simulink model "Grua_MC_R2_Ciclo_Completo_SFC"  (R2025b)
settings: Solver=ode23t  StartTime=0.0  StopTime=640  MaxStep=T_s  RelTol=1e-4
InitFcn:
  | addpath(fileparts(get_param(bdroot,'FileName')),'-begin');
  | run(fullfile(fileparts(get_param(bdroot,'FileName')),'definir_buses_variadores.m'));
  | run(fullfile(fileparts(get_param(bdroot,'FileName')),'parametros_ganancias_cascada_29072026.m'));
  | run(fullfile(fileparts(get_param(bdroot,'FileName')),'configurar_modelo_final_hmi.m'));
  | run(fullfile(fileparts(get_param(bdroot,'FileName')),'configurar_parametros_variadores.m'));
  | Pvis.Ts_viz=.04;Pvis.enable=true;Pvis.keepFigureOnTerminate=true;Pvis.hmi.fastDiagnostic=false;
undefined symbols (not defined in the file or in its folder): b_cx, b_cy, b_hb, b_hEb, b_heq, b_t, b_tb, b_teq, b_tw, b_wu, g, H_c, HMI, i_h, i_t, J_heq, J_teq, K_cy, K_tw, k_wu, L_h0, l_hi, M_c_profile, M_s, M_t, MC_FF, nLevels0, omega_hmRATED, r_hd, r_td, slotBlock, T_hbMax, T_hEbMax, T_hmMax, T_s, T_s1, T_tbMax, T_tmMax, tau_hm, tau_tm, traj_duration, traj_x_start, traj_x_target, v_hmaxLoaded, v_hmaxUnloaded, x_tmax, x_tmin, Y_c0, Y_t0, Zbase
libraries: simulink x1, aerolibanimutils x1
(part 2 of 4)

== system Grua_MC_R2_Ciclo_Completo_SFC/Actualizar_Yc ==
  tipo_evento : Inport
  slot_evento : Inport  Port=2
  Trigger : TriggerPort  VariantControl=(inherit)  PortDimensions=1
  Constant : Constant  Value=Zbase
  Constant1 : Constant  Value=slotBlock
  Constant2 : Constant  Value=H_c
  Unit Delay : UnitDelay  InitialCondition=nLevels0  SampleTime=-1  HasFrameUpgradeWarning=on
  update_perfil_std : MATLAB Function  TreatAsAtomicUnit=on
  Y_c : Outport  InitialOutput=Y_c0
  wires:
  update_perfil_std/2(Y_c) -> Y_c/1
  slot_evento/1 -> update_perfil_std/3(slot_evento)
  update_perfil_std/1(nLevels_new) -> Unit Delay/1
  tipo_evento/1 -> update_perfil_std/2(tipo_evento)
  Unit Delay/1 -> update_perfil_std/1(nLevels)
  Constant/1 -> update_perfil_std/4(Zbase)
  Constant1/1 -> update_perfil_std/5(slotBlock)
  Constant2/1 -> update_perfil_std/6(h_std)

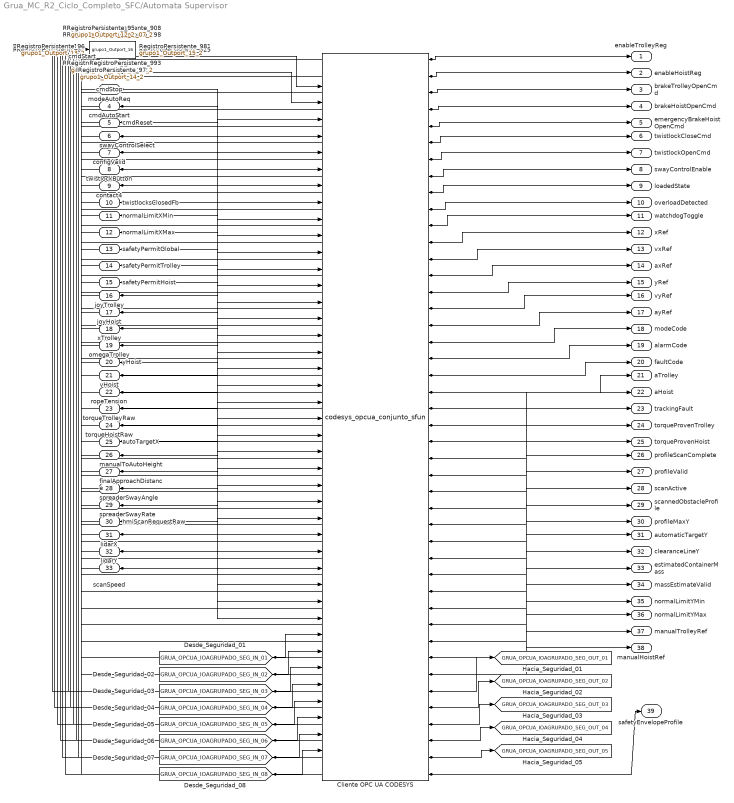
== system Grua_MC_R2_Ciclo_Completo_SFC/Automata Supervisor ==
  cmdStart : Inport
  cmdStop : Inport  Port=2
  modeAutoReq : Inport  Port=3
  cmdAutoStart : Inport  Port=4
  cmdReset : Inport  Port=5
  swayControlSelect : Inport  Port=6
  configValid : Inport  Port=7
  twistlockButton : Inport  Port=8
  contact4 : Inport  Port=9
  twistlocksClosedFb : Inport  Port=10
  normalLimitXMin : Inport  Port=11
  normalLimitXMax : Inport  Port=12
  safetyPermitGlobal : Inport  Port=13
  safetyPermitTrolley : Inport  Port=14
  safetyPermitHoist : Inport  Port=15
  joyTrolley : Inport  Port=16
  joyHoist : Inport  Port=17
  xTrolley : Inport  Port=18
  omegaTrolley : Inport  Port=19
  yHoist : Inport  Port=20
  vHoist : Inport  Port=21
  ropeTension : Inport  Port=22
  torqueTrolleyRaw : Inport  Port=23
  torqueHoistRaw : Inport  Port=24
  autoTargetX : Inport  Port=25
  manualToAutoHeight : Inport  Port=26
  finalApproachDistance : Inport  Port=27
  spreaderSwayAngle : Inport  Port=28
  spreaderSwayRate : Inport  Port=29
  hmiScanRequestRaw : Inport  Port=30
  lidarX : Inport  Port=31
  lidarY : Inport  Port=32
  scanSpeed : Inport  Port=33
  Cliente OPC UA CODESYS : M-S-Function  FunctionName=codesys_opcua_conjunto_sfun
  RegistroPersistente_100 : ToWorkspace  VariableName=grupo1_Outport_17  SaveFormat=Timeseries  SampleTime=-1
      settings: Decimation=10
  RegistroPersistente_101 : ToWorkspace  VariableName=grupo1_Outport_18_2  SaveFormat=Timeseries  SampleTime=-1
      settings: Decimation=10
  RegistroPersistente_102 : ToWorkspace  VariableName=grupo1_Outport_19_2  SaveFormat=Timeseries  SampleTime=-1
      settings: Decimation=10
  RegistroPersistente_103 : ToWorkspace  VariableName=grupo1_Outport_20_2  SaveFormat=Timeseries  SampleTime=-1
      settings: Decimation=10
  RegistroPersistente_104 : ToWorkspace  VariableName=grupo1_Outport_21_2  SaveFormat=Timeseries  SampleTime=-1
      settings: Decimation=10
  RegistroPersistente_105 : ToWorkspace  VariableName=grupo1_Outport_22_2  SaveFormat=Timeseries  SampleTime=-1
      settings: Decimation=10
  RegistroPersistente_106 : ToWorkspace  VariableName=grupo1_Outport_23_2  SaveFormat=Timeseries  SampleTime=-1
      settings: Decimation=10
  RegistroPersistente_107 : ToWorkspace  VariableName=grupo1_Outport_24_2  SaveFormat=Timeseries  SampleTime=-1
      settings: Decimation=10
  RegistroPersistente_108 : ToWorkspace  VariableName=grupo1_Outport_25_2  SaveFormat=Timeseries  SampleTime=-1
      settings: Decimation=10
  RegistroPersistente_109 : ToWorkspace  VariableName=grupo1_Outport_26_2  SaveFormat=Timeseries  SampleTime=-1
      settings: Decimation=10
  RegistroPersistente_110 : ToWorkspace  VariableName=grupo1_Outport_27_2  SaveFormat=Timeseries  SampleTime=-1
      settings: Decimation=10
  RegistroPersistente_111 : ToWorkspace  VariableName=grupo1_Outport_28_2  SaveFormat=Timeseries  SampleTime=-1
      settings: Decimation=10
  RegistroPersistente_112 : ToWorkspace  VariableName=grupo1_Outport_29_2  SaveFormat=Timeseries  SampleTime=-1
      settings: Decimation=10
  RegistroPersistente_113 : ToWorkspace  VariableName=grupo1_Outport_30_2  SaveFormat=Timeseries  SampleTime=-1
      settings: Decimation=10
  RegistroPersistente_114 : ToWorkspace  VariableName=grupo1_Outport_31_2  SaveFormat=Timeseries  SampleTime=-1
      settings: Decimation=10
  RegistroPersistente_115 : ToWorkspace  VariableName=grupo1_Outport_32_2  SaveFormat=Timeseries  SampleTime=-1
      settings: Decimation=10
  RegistroPersistente_116 : ToWorkspace  VariableName=grupo1_Outport_33_2  SaveFormat=Timeseries  SampleTime=-1
      settings: Decimation=10
  RegistroPersistente_117 : ToWorkspace  VariableName=grupo1_Outport_34_2  SaveFormat=Timeseries  SampleTime=-1
      settings: Decimation=10
  RegistroPersistente_118 : ToWorkspace  VariableName=grupo1_Outport_35_2  SaveFormat=Timeseries  SampleTime=-1
      settings: Decimation=10
  RegistroPersistente_119 : ToWorkspace  VariableName=grupo1_Outport_36_2  SaveFormat=Timeseries  SampleTime=-1
      settings: Decimation=10
  RegistroPersistente_120 : ToWorkspace  VariableName=grupo1_Outport_37_2  SaveFormat=Timeseries  SampleTime=-1
      settings: Decimation=10
  RegistroPersistente_121 : ToWorkspace  VariableName=grupo1_Outport_38_2  SaveFormat=Timeseries  SampleTime=-1
      settings: Decimation=10
  RegistroPersistente_122 : ToWorkspace  VariableName=grupo1_Outport_39  SaveFormat=Timeseries  SampleTime=-1
      settings: Decimation=10
  RegistroPersistente_123 : ToWorkspace  VariableName=grupo1_Outport_40  SaveFormat=Timeseries  SampleTime=-1
      settings: Decimation=10
  RegistroPersistente_124 : ToWorkspace  VariableName=grupo1_Outport_41  SaveFormat=Timeseries  SampleTime=-1
      settings: Decimation=10
  RegistroPersistente_125 : ToWorkspace  VariableName=grupo1_Outport_42  SaveFormat=Timeseries  SampleTime=-1
      settings: Decimation=10
  RegistroPersistente_126 : ToWorkspace  VariableName=grupo1_Outport_43  SaveFormat=Timeseries  SampleTime=-1
      settings: Decimation=10
  RegistroPersistente_127 : ToWorkspace  VariableName=grupo1_Outport_44  SaveFormat=Timeseries  SampleTime=-1
      settings: Decimation=10
  RegistroPersistente_128 : ToWorkspace  VariableName=grupo1_Inport_34  SaveFormat=Timeseries  SampleTime=-1
      settings: Decimation=10
  RegistroPersistente_129 : ToWorkspace  VariableName=grupo1_Inport_35  SaveFormat=Timeseries  SampleTime=-1
      settings: Decimation=10
  RegistroPersistente_130 : ToWorkspace  VariableName=grupo1_Inport_36  SaveFormat=Timeseries  SampleTime=-1
      settings: Decimation=10
  RegistroPersistente_131 : ToWorkspace  VariableName=grupo1_Inport_37  SaveFormat=Timeseries  SampleTime=-1
      settings: Decimation=10
  RegistroPersistente_132 : ToWorkspace  VariableName=grupo1_Inport_38  SaveFormat=Timeseries  SampleTime=-1
      settings: Decimation=10
  RegistroPersistente_133 : ToWorkspace  VariableName=grupo1_Inport_39  SaveFormat=Timeseries  SampleTime=-1
      settings: Decimation=10
  RegistroPersistente_134 : ToWorkspace  VariableName=grupo1_Inport_40  SaveFormat=Timeseries  SampleTime=-1
      settings: Decimation=10
  RegistroPersistente_135 : ToWorkspace  VariableName=grupo1_Inport_41  SaveFormat=Timeseries  SampleTime=-1
      settings: Decimation=10
  RegistroPersistente_51 : ToWorkspace  VariableName=grupo1_Inport_01_2  SaveFormat=Timeseries  SampleTime=-1
      settings: Decimation=10
  RegistroPersistente_52 : ToWorkspace  VariableName=grupo1_Inport_02_2  SaveFormat=Timeseries  SampleTime=-1
      settings: Decimation=10
  RegistroPersistente_53 : ToWorkspace  VariableName=grupo1_Inport_03_2  SaveFormat=Timeseries  SampleTime=-1
      settings: Decimation=10
  RegistroPersistente_54 : ToWorkspace  VariableName=grupo1_Inport_04_2  SaveFormat=Timeseries  SampleTime=-1
      settings: Decimation=10
  RegistroPersistente_55 : ToWorkspace  VariableName=grupo1_Inport_05_2  SaveFormat=Timeseries  SampleTime=-1
      settings: Decimation=10
  RegistroPersistente_56 : ToWorkspace  VariableName=grupo1_Inport_06_2  SaveFormat=Timeseries  SampleTime=-1
      settings: Decimation=10
  RegistroPersistente_57 : ToWorkspace  VariableName=grupo1_Inport_07_2  SaveFormat=Timeseries  SampleTime=-1
      settings: Decimation=10
  RegistroPersistente_58 : ToWorkspace  VariableName=grupo1_Inport_08_2  SaveFormat=Timeseries  SampleTime=-1
      settings: Decimation=10
  RegistroPersistente_59 : ToWorkspace  VariableName=grupo1_Inport_09_2  SaveFormat=Timeseries  SampleTime=-1
      settings: Decimation=10
  RegistroPersistente_60 : ToWorkspace  VariableName=grupo1_Inport_10_2  SaveFormat=Timeseries  SampleTime=-1
      settings: Decimation=10
  RegistroPersistente_61 : ToWorkspace  VariableName=grupo1_Inport_11_2  SaveFormat=Timeseries  SampleTime=-1
      settings: Decimation=10
  RegistroPersistente_62 : ToWorkspace  VariableName=grupo1_Inport_12_2  SaveFormat=Timeseries  SampleTime=-1
      settings: Decimation=10
  RegistroPersistente_63 : ToWorkspace  VariableName=grupo1_Inport_13_2  SaveFormat=Timeseries  SampleTime=-1
      settings: Decimation=10
  RegistroPersistente_64 : ToWorkspace  VariableName=grupo1_Inport_14_2  SaveFormat=Timeseries  SampleTime=-1
      settings: Decimation=10
  RegistroPersistente_65 : ToWorkspace  VariableName=grupo1_Inport_15_2  SaveFormat=Timeseries  SampleTime=-1
      settings: Decimation=10
  RegistroPersistente_66 : ToWorkspace  VariableName=grupo1_Inport_16_2  SaveFormat=Timeseries  SampleTime=-1
      settings: Decimation=10
  RegistroPersistente_67 : ToWorkspace  VariableName=grupo1_Inport_17_2  SaveFormat=Timeseries  SampleTime=-1
      settings: Decimation=10
  RegistroPersistente_68 : ToWorkspace  VariableName=grupo1_Inport_18_2  SaveFormat=Timeseries  SampleTime=-1
      settings: Decimation=10
  RegistroPersistente_69 : ToWorkspace  VariableName=grupo1_Inport_19_2  SaveFormat=Timeseries  SampleTime=-1
      settings: Decimation=10
  RegistroPersistente_70 : ToWorkspace  VariableName=grupo1_Inport_20_2  SaveFormat=Timeseries  SampleTime=-1
      settings: Decimation=10
  RegistroPersistente_71 : ToWorkspace  VariableName=grupo1_Inport_21_2  SaveFormat=Timeseries  SampleTime=-1
      settings: Decimation=10
  RegistroPersistente_72 : ToWorkspace  VariableName=grupo1_Inport_22_2  SaveFormat=Timeseries  SampleTime=-1
      settings: Decimation=10
  RegistroPersistente_73 : ToWorkspace  VariableName=grupo1_Inport_23_2  SaveFormat=Timeseries  SampleTime=-1
      settings: Decimation=10
  RegistroPersistente_74 : ToWorkspace  VariableName=grupo1_Inport_24_2  SaveFormat=Timeseries  SampleTime=-1
      settings: Decimation=10
  RegistroPersistente_75 : ToWorkspace  VariableName=grupo1_Inport_25_2  SaveFormat=Timeseries  SampleTime=-1
      settings: Decimation=10
  RegistroPersistente_76 : ToWorkspace  VariableName=grupo1_Inport_26_2  SaveFormat=Timeseries  SampleTime=-1
      settings: Decimation=10
  RegistroPersistente_77 : ToWorkspace  VariableName=grupo1_Inport_27_2  SaveFormat=Timeseries  SampleTime=-1
      settings: Decimation=10
  RegistroPersistente_78 : ToWorkspace  VariableName=grupo1_Inport_28_2  SaveFormat=Timeseries  SampleTime=-1
      settings: Decimation=10
  RegistroPersistente_79 : ToWorkspace  VariableName=grupo1_Inport_29_2  SaveFormat=Timeseries  SampleTime=-1
      settings: Decimation=10
  RegistroPersistente_80 : ToWorkspace  VariableName=grupo1_Inport_30_2  SaveFormat=Timeseries  SampleTime=-1
      settings: Decimation=10
  RegistroPersistente_81 : ToWorkspace  VariableName=grupo1_Inport_31_2  SaveFormat=Timeseries  SampleTime=-1
      settings: Decimation=10
  RegistroPersistente_82 : ToWorkspace  VariableName=grupo1_Inport_32_2  SaveFormat=Timeseries  SampleTime=-1
      settings: Decimation=10
  RegistroPersistente_83 : ToWorkspace  VariableName=grupo1_Inport_33_2  SaveFormat=Timeseries  SampleTime=-1
      settings: Decimation=10
  RegistroPersistente_84 : ToWorkspace  VariableName=grupo1_Outport_01_2  SaveFormat=Timeseries  SampleTime=-1
      settings: Decimation=10
  RegistroPersistente_85 : ToWorkspace  VariableName=grupo1_Outport_02_2  SaveFormat=Timeseries  SampleTime=-1
      settings: Decimation=10
  RegistroPersistente_86 : ToWorkspace  VariableName=grupo1_Outport_03  SaveFormat=Timeseries  SampleTime=-1
      settings: Decimation=10
  RegistroPersistente_87 : ToWorkspace  VariableName=grupo1_Outport_04_2  SaveFormat=Timeseries  SampleTime=-1
      settings: Decimation=10
  RegistroPersistente_88 : ToWorkspace  VariableName=grupo1_Outport_05_2  SaveFormat=Timeseries  SampleTime=-1
      settings: Decimation=10
  RegistroPersistente_89 : ToWorkspace  VariableName=grupo1_Outport_06_2  SaveFormat=Timeseries  SampleTime=-1
      settings: Decimation=10
  RegistroPersistente_90 : ToWorkspace  VariableName=grupo1_Outport_07_2  SaveFormat=Timeseries  SampleTime=-1
      settings: Decimation=10
  RegistroPersistente_91 : ToWorkspace  VariableName=grupo1_Outport_08  SaveFormat=Timeseries  SampleTime=-1
      settings: Decimation=10
  RegistroPersistente_92 : ToWorkspace  VariableName=grupo1_Outport_09_2  SaveFormat=Timeseries  SampleTime=-1
      settings: Decimation=10
  RegistroPersistente_93 : ToWorkspace  VariableName=grupo1_Outport_10_2  SaveFormat=Timeseries  SampleTime=-1
      settings: Decimation=10
  RegistroPersistente_94 : ToWorkspace  VariableName=grupo1_Outport_11_2  SaveFormat=Timeseries  SampleTime=-1
      settings: Decimation=10
  RegistroPersistente_95 : ToWorkspace  VariableName=grupo1_Outport_12_2  SaveFormat=Timeseries  SampleTime=-1
      settings: Decimation=10
  RegistroPersistente_96 : ToWorkspace  VariableName=grupo1_Outport_13_2  SaveFormat=Timeseries  SampleTime=-1
      settings: Decimation=10
  RegistroPersistente_97 : ToWorkspace  VariableName=grupo1_Outport_14_2  SaveFormat=Timeseries  SampleTime=-1
      settings: Decimation=10
  RegistroPersistente_98 : ToWorkspace  VariableName=grupo1_Outport_15_2  SaveFormat=Timeseries  SampleTime=-1
      settings: Decimation=10
  RegistroPersistente_99 : ToWorkspace  VariableName=grupo1_Outport_16  SaveFormat=Timeseries  SampleTime=-1
      settings: Decimation=10
  enableTrolleyReg : Outport
  enableHoistReg : Outport  Port=2
  brakeTrolleyOpenCmd : Outport  Port=3
  brakeHoistOpenCmd : Outport  Port=4
  emergencyBrakeHoistOpenCmd : Outport  Port=5
  twistlockCloseCmd : Outport  Port=6
  twistlockOpenCmd : Outport  Port=7
  swayControlEnable : Outport  Port=8
  loadedState : Outport  Port=9
  overloadDetected : Outport  Port=10
  watchdogToggle : Outport  Port=11
  xRef : Outport  Port=12
  vxRef : Outport  Port=13
  axRef : Outport  Port=14
  yRef : Outport  Port=15
  vyRef : Outport  Port=16
  ayRef : Outport  Port=17
  modeCode : Outport  Port=18
  alarmCode : Outport  Port=19
  faultCode : Outport  Port=20
  aTrolley : Outport  Port=21
  aHoist : Outport  Port=22
  trackingFault : Outport  Port=23
  torqueProvenTrolley : Outport  Port=24
  torqueProvenHoist : Outport  Port=25
  profileScanComplete : Outport  Port=26
  profileValid : Outport  Port=27
  scanActive : Outport  Port=28
  scannedObstacleProfile : Outport  Port=29
  profileMaxY : Outport  Port=30
  automaticTargetY : Outport  Port=31
  clearanceLineY : Outport  Port=32
  estimatedContainerMass : Outport  Port=33
  massEstimateValid : Outport  Port=34
  normalLimitYMin : Outport  Port=35
  normalLimitYMax : Outport  Port=36
  manualTrolleyRef : Outport  Port=37
  manualHoistRef : Outport  Port=38
  safetyEnvelopeProfile : Outport  Port=39
  tag scope: GRUA_OPCUA_IOAGRUPADO_SEG_OUT_01=global, GRUA_OPCUA_IOAGRUPADO_SEG_OUT_02=global, GRUA_OPCUA_IOAGRUPADO_SEG_OUT_03=global, GRUA_OPCUA_IOAGRUPADO_SEG_OUT_04=global, GRUA_OPCUA_IOAGRUPADO_SEG_OUT_05=global
  wires:
  Cliente OPC UA CODESYS/44 -> safetyEnvelopeProfile/1, RegistroPersistente_127/1
  Cliente OPC UA CODESYS/43 -> [GRUA_OPCUA_IOAGRUPADO_SEG_OUT_05], RegistroPersistente_126/1
  Cliente OPC UA CODESYS/42 -> [GRUA_OPCUA_IOAGRUPADO_SEG_OUT_04], RegistroPersistente_125/1
  Cliente OPC UA CODESYS/41 -> [GRUA_OPCUA_IOAGRUPADO_SEG_OUT_03], RegistroPersistente_124/1
  Cliente OPC UA CODESYS/40 -> [GRUA_OPCUA_IOAGRUPADO_SEG_OUT_02], RegistroPersistente_123/1
  Cliente OPC UA CODESYS/39 -> [GRUA_OPCUA_IOAGRUPADO_SEG_OUT_01], RegistroPersistente_122/1
  [GRUA_OPCUA_IOAGRUPADO_SEG_IN_08] -> Cliente OPC UA CODESYS/41, RegistroPersistente_135/1
  [GRUA_OPCUA_IOAGRUPADO_SEG_IN_07] -> Cliente OPC UA CODESYS/40, RegistroPersistente_134/1
  [GRUA_OPCUA_IOAGRUPADO_SEG_IN_06] -> Cliente OPC UA CODESYS/39, RegistroPersistente_133/1
  [GRUA_OPCUA_IOAGRUPADO_SEG_IN_05] -> Cliente OPC UA CODESYS/38, RegistroPersistente_132/1
  [GRUA_OPCUA_IOAGRUPADO_SEG_IN_04] -> Cliente OPC UA CODESYS/37, RegistroPersistente_131/1
  [GRUA_OPCUA_IOAGRUPADO_SEG_IN_03] -> Cliente OPC UA CODESYS/36, RegistroPersistente_130/1
  [GRUA_OPCUA_IOAGRUPADO_SEG_IN_02] -> Cliente OPC UA CODESYS/35, RegistroPersistente_129/1
  [GRUA_OPCUA_IOAGRUPADO_SEG_IN_01] -> Cliente OPC UA CODESYS/34, RegistroPersistente_128/1
  Cliente OPC UA CODESYS/38 -> manualHoistRef/1, RegistroPersistente_121/1
  Cliente OPC UA CODESYS/37 -> manualTrolleyRef/1, RegistroPersistente_120/1
  Cliente OPC UA CODESYS/36 -> normalLimitYMax/1, RegistroPersistente_119/1
  Cliente OPC UA CODESYS/35 -> normalLimitYMin/1, RegistroPersistente_118/1
  Cliente OPC UA CODESYS/34 -> massEstimateValid/1, RegistroPersistente_117/1
  Cliente OPC UA CODESYS/33 -> estimatedContainerMass/1, RegistroPersistente_116/1
  Cliente OPC UA CODESYS/32 -> clearanceLineY/1, RegistroPersistente_115/1
  Cliente OPC UA CODESYS/31 -> automaticTargetY/1, RegistroPersistente_114/1
  Cliente OPC UA CODESYS/30 -> profileMaxY/1, RegistroPersistente_113/1
  Cliente OPC UA CODESYS/29 -> scannedObstacleProfile/1, RegistroPersistente_112/1
  Cliente OPC UA CODESYS/28 -> scanActive/1, RegistroPersistente_111/1
  Cliente OPC UA CODESYS/27 -> profileValid/1, RegistroPersistente_110/1
  Cliente OPC UA CODESYS/26 -> profileScanComplete/1, RegistroPersistente_109/1
  Cliente OPC UA CODESYS/25 -> torqueProvenHoist/1, RegistroPersistente_108/1
  Cliente OPC UA CODESYS/24 -> torqueProvenTrolley/1, RegistroPersistente_107/1
  Cliente OPC UA CODESYS/23 -> trackingFault/1, RegistroPersistente_106/1
  Cliente OPC UA CODESYS/22 -> aHoist/1, RegistroPersistente_105/1
  Cliente OPC UA CODESYS/21 -> aTrolley/1, RegistroPersistente_104/1
  Cliente OPC UA CODESYS/20 -> faultCode/1, RegistroPersistente_103/1
  Cliente OPC UA CODESYS/19 -> alarmCode/1, RegistroPersistente_102/1
  Cliente OPC UA CODESYS/18 -> modeCode/1, RegistroPersistente_101/1
  Cliente OPC UA CODESYS/17 -> ayRef/1, RegistroPersistente_100/1
  Cliente OPC UA CODESYS/16 -> vyRef/1, RegistroPersistente_99/1
  Cliente OPC UA CODESYS/15 -> yRef/1, RegistroPersistente_98/1
  Cliente OPC UA CODESYS/14 -> axRef/1, RegistroPersistente_97/1
  Cliente OPC UA CODESYS/13 -> vxRef/1, RegistroPersistente_96/1
  Cliente OPC UA CODESYS/12 -> xRef/1, RegistroPersistente_95/1
  Cliente OPC UA CODESYS/11 -> watchdogToggle/1, RegistroPersistente_94/1
  Cliente OPC UA CODESYS/10 -> overloadDetected/1, RegistroPersistente_93/1
  Cliente OPC UA CODESYS/9 -> loadedState/1, RegistroPersistente_92/1
  Cliente OPC UA CODESYS/8 -> swayControlEnable/1, RegistroPersistente_91/1
  Cliente OPC UA CODESYS/7 -> twistlockOpenCmd/1, RegistroPersistente_90/1
  Cliente OPC UA CODESYS/6 -> twistlockCloseCmd/1, RegistroPersistente_89/1
  Cliente OPC UA CODESYS/5 -> emergencyBrakeHoistOpenCmd/1, RegistroPersistente_88/1
  Cliente OPC UA CODESYS/4 -> brakeHoistOpenCmd/1, RegistroPersistente_87/1
  Cliente OPC UA CODESYS/3 -> brakeTrolleyOpenCmd/1, RegistroPersistente_86/1
  Cliente OPC UA CODESYS/2 -> enableHoistReg/1, RegistroPersistente_85/1
  Cliente OPC UA CODESYS/1 -> enableTrolleyReg/1, RegistroPersistente_84/1
  scanSpeed/1 -> Cliente OPC UA CODESYS/33, RegistroPersistente_83/1
  lidarY/1 -> Cliente OPC UA CODESYS/32, RegistroPersistente_82/1
  lidarX/1 -> Cliente OPC UA CODESYS/31, RegistroPersistente_81/1
  hmiScanRequestRaw/1 -> Cliente OPC UA CODESYS/30, RegistroPersistente_80/1
  spreaderSwayRate/1 -> Cliente OPC UA CODESYS/29, RegistroPersistente_79/1
  spreaderSwayAngle/1 -> Cliente OPC UA CODESYS/28, RegistroPersistente_78/1
  finalApproachDistance/1 -> Cliente OPC UA CODESYS/27, RegistroPersistente_77/1
  manualToAutoHeight/1 -> Cliente OPC UA CODESYS/26, RegistroPersistente_76/1
  autoTargetX/1 -> Cliente OPC UA CODESYS/25, RegistroPersistente_75/1
  torqueHoistRaw/1 -> Cliente OPC UA CODESYS/24, RegistroPersistente_74/1
  torqueTrolleyRaw/1 -> Cliente OPC UA CODESYS/23, RegistroPersistente_73/1
  ropeTension/1 -> Cliente OPC UA CODESYS/22, RegistroPersistente_72/1
  vHoist/1 -> Cliente OPC UA CODESYS/21, RegistroPersistente_71/1
  yHoist/1 -> Cliente OPC UA CODESYS/20, RegistroPersistente_70/1
  omegaTrolley/1 -> Cliente OPC UA CODESYS/19, RegistroPersistente_69/1
  xTrolley/1 -> Cliente OPC UA CODESYS/18, RegistroPersistente_68/1
  joyHoist/1 -> Cliente OPC UA CODESYS/17, RegistroPersistente_67/1
  joyTrolley/1 -> Cliente OPC UA CODESYS/16, RegistroPersistente_66/1
  safetyPermitHoist/1 -> Cliente OPC UA CODESYS/15, RegistroPersistente_65/1
  safetyPermitTrolley/1 -> Cliente OPC UA CODESYS/14, RegistroPersistente_64/1
  safetyPermitGlobal/1 -> Cliente OPC UA CODESYS/13, RegistroPersistente_63/1
  normalLimitXMax/1 -> Cliente OPC UA CODESYS/12, RegistroPersistente_62/1
  normalLimitXMin/1 -> Cliente OPC UA CODESYS/11, RegistroPersistente_61/1
  twistlocksClosedFb/1 -> Cliente OPC UA CODESYS/10, RegistroPersistente_60/1
  contact4/1 -> Cliente OPC UA CODESYS/9, RegistroPersistente_59/1
  twistlockButton/1 -> Cliente OPC UA CODESYS/8, RegistroPersistente_58/1
  configValid/1 -> Cliente OPC UA CODESYS/7, RegistroPersistente_57/1
  swayControlSelect/1 -> Cliente OPC UA CODESYS/6, RegistroPersistente_56/1
  cmdReset/1 -> Cliente OPC UA CODESYS/5, RegistroPersistente_55/1
  cmdAutoStart/1 -> Cliente OPC UA CODESYS/4, RegistroPersistente_54/1
  modeAutoReq/1 -> Cliente OPC UA CODESYS/3, RegistroPersistente_53/1
  cmdStop/1 -> Cliente OPC UA CODESYS/2, RegistroPersistente_52/1
  cmdStart/1 -> Cliente OPC UA CODESYS/1, RegistroPersistente_51/1

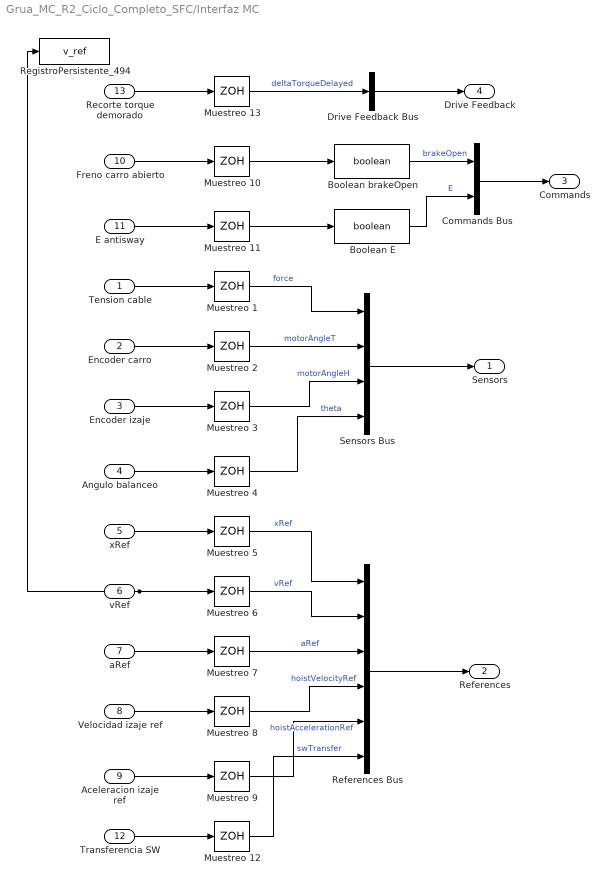
== system Grua_MC_R2_Ciclo_Completo_SFC/Interfaz MC ==
  Tension cable : Inport
  Encoder carro : Inport  Port=2
  Encoder izaje : Inport  Port=3
  Angulo balanceo : Inport  Port=4
  xRef : Inport  Port=5
  vRef : Inport  Port=6
  aRef : Inport  Port=7
  Velocidad izaje ref : Inport  Port=8
  Aceleracion izaje ref : Inport  Port=9
  Freno carro abierto : Inport  Port=10
  E antisway : Inport  Port=11
  Transferencia SW : Inport  Port=12
  Recorte torque demorado : Inport  Port=13
  Boolean E : DataTypeConversion  OutDataTypeStr=boolean  SaturateOnIntegerOverflow=off  RndMeth=Floor
  Boolean brakeOpen : DataTypeConversion  OutDataTypeStr=boolean  SaturateOnIntegerOverflow=off  RndMeth=Floor
  Commands Bus : BusCreator  Inputs=2  OutDataTypeStr=Bus: MCFF_Commands  NonVirtualBus=on
  Drive Feedback Bus : BusCreator  Inputs=1  OutDataTypeStr=Bus: MCFF_DriveFeedback  NonVirtualBus=on
  Muestreo {1..13} (13 alike) : ZeroOrderHold  SampleTime=T_s
  References Bus : BusCreator  Inputs=6  OutDataTypeStr=Bus: MCFF_References  NonVirtualBus=on
  RegistroPersistente_494 : ToWorkspace  VariableName=v_ref  SaveFormat=Timeseries  SampleTime=-1
      settings: Decimation=10
  Sensors Bus : BusCreator  Inputs=4  OutDataTypeStr=Bus: MCFF_Sensors  NonVirtualBus=on
  Sensors : Outport
  References : Outport  Port=2
  Commands : Outport  Port=3
  Drive Feedback : Outport  Port=4
  wires:
  Drive Feedback Bus/1 -> Drive Feedback/1
  Muestreo 4/1 -> Sensors Bus/4  "theta"
  E antisway/1 -> Muestreo 11/1
  Recorte torque demorado/1 -> Muestreo 13/1
  Encoder carro/1 -> Muestreo 2/1
  Tension cable/1 -> Muestreo 1/1
  Muestreo 3/1 -> Sensors Bus/3  "motorAngleH"
  Freno carro abierto/1 -> Muestreo 10/1
  xRef/1 -> Muestreo 5/1
  Angulo balanceo/1 -> Muestreo 4/1
  Muestreo 11/1 -> Boolean E/1
  Encoder izaje/1 -> Muestreo 3/1
  Commands Bus/1 -> Commands/1
  vRef/1 -> Muestreo 6/1, RegistroPersistente_494/1
  Boolean E/1 -> Commands Bus/2  "E"
  aRef/1 -> Muestreo 7/1
  Velocidad izaje ref/1 -> Muestreo 8/1
  Aceleracion izaje ref/1 -> Muestreo 9/1
  Transferencia SW/1 -> Muestreo 12/1
  Muestreo 13/1 -> Drive Feedback Bus/1  "deltaTorqueDelayed"
  Muestreo 10/1 -> Boolean brakeOpen/1
  Muestreo 1/1 -> Sensors Bus/1  "force"
  Muestreo 2/1 -> Sensors Bus/2  "motorAngleT"
  Muestreo 5/1 -> References Bus/1  "xRef"
  Muestreo 6/1 -> References Bus/2  "vRef"
  Muestreo 7/1 -> References Bus/3  "aRef"
  Muestreo 8/1 -> References Bus/4  "hoistVelocityRef"
  Muestreo 9/1 -> References Bus/5  "hoistAccelerationRef"
  Muestreo 12/1 -> References Bus/6  "swTransfer"
  Boolean brakeOpen/1 -> Commands Bus/1  "brakeOpen"
  Sensors Bus/1 -> Sensors/1
  References Bus/1 -> References/1

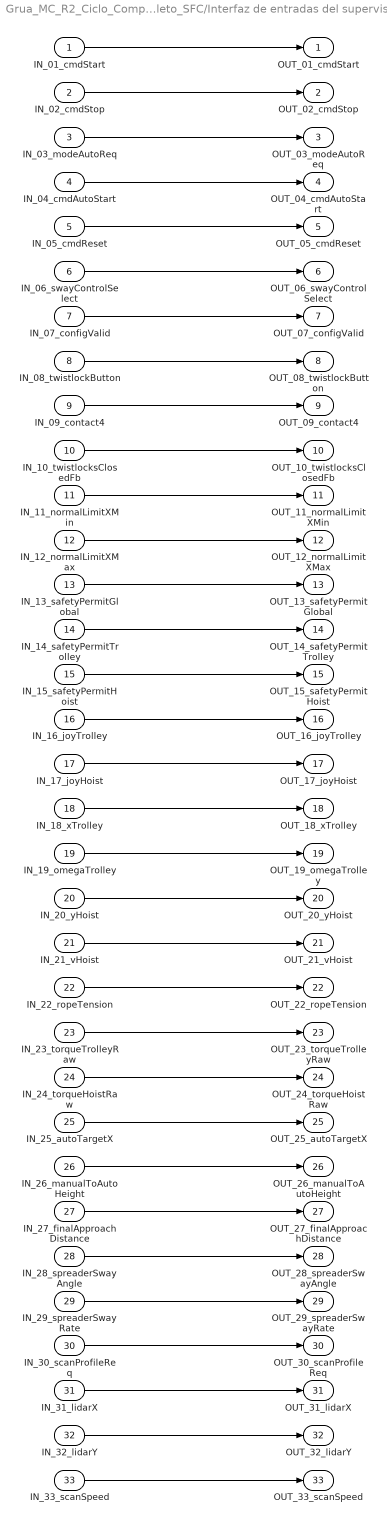
== system Grua_MC_R2_Ciclo_Completo_SFC/Interfaz de entradas del supervisor ==
  IN_01_cmdStart : Inport
  IN_02_cmdStop : Inport  Port=2
  IN_03_modeAutoReq : Inport  Port=3
  IN_04_cmdAutoStart : Inport  Port=4
  IN_05_cmdReset : Inport  Port=5
  IN_06_swayControlSelect : Inport  Port=6
  IN_07_configValid : Inport  Port=7
  IN_08_twistlockButton : Inport  Port=8
  IN_09_contact4 : Inport  Port=9
  IN_10_twistlocksClosedFb : Inport  Port=10
  IN_11_normalLimitXMin : Inport  Port=11
  IN_12_normalLimitXMax : Inport  Port=12
  IN_13_safetyPermitGlobal : Inport  Port=13
  IN_14_safetyPermitTrolley : Inport  Port=14
  IN_15_safetyPermitHoist : Inport  Port=15
  IN_16_joyTrolley : Inport  Port=16
  IN_17_joyHoist : Inport  Port=17
  IN_18_xTrolley : Inport  Port=18
  IN_19_omegaTrolley : Inport  Port=19
  IN_20_yHoist : Inport  Port=20
  IN_21_vHoist : Inport  Port=21
  IN_22_ropeTension : Inport  Port=22
  IN_23_torqueTrolleyRaw : Inport  Port=23
  IN_24_torqueHoistRaw : Inport  Port=24
  IN_25_autoTargetX : Inport  Port=25
  IN_26_manualToAutoHeight : Inport  Port=26
  IN_27_finalApproachDistance : Inport  Port=27
  IN_28_spreaderSwayAngle : Inport  Port=28
  IN_29_spreaderSwayRate : Inport  Port=29
  IN_30_scanProfileReq : Inport  Port=30
  IN_31_lidarX : Inport  Port=31
  IN_32_lidarY : Inport  Port=32
  IN_33_scanSpeed : Inport  Port=33
  OUT_01_cmdStart : Outport
  OUT_02_cmdStop : Outport  Port=2
  OUT_03_modeAutoReq : Outport  Port=3
  OUT_04_cmdAutoStart : Outport  Port=4
  OUT_05_cmdReset : Outport  Port=5
  OUT_06_swayControlSelect : Outport  Port=6
  OUT_07_configValid : Outport  Port=7
  OUT_08_twistlockButton : Outport  Port=8
  OUT_09_contact4 : Outport  Port=9
  OUT_10_twistlocksClosedFb : Outport  Port=10
  OUT_11_normalLimitXMin : Outport  Port=11
  OUT_12_normalLimitXMax : Outport  Port=12
  OUT_13_safetyPermitGlobal : Outport  Port=13
  OUT_14_safetyPermitTrolley : Outport  Port=14
  OUT_15_safetyPermitHoist : Outport  Port=15
  OUT_16_joyTrolley : Outport  Port=16
  OUT_17_joyHoist : Outport  Port=17
  OUT_18_xTrolley : Outport  Port=18
  OUT_19_omegaTrolley : Outport  Port=19
  OUT_20_yHoist : Outport  Port=20
  OUT_21_vHoist : Outport  Port=21
  OUT_22_ropeTension : Outport  Port=22
  OUT_23_torqueTrolleyRaw : Outport  Port=23
  OUT_24_torqueHoistRaw : Outport  Port=24
  OUT_25_autoTargetX : Outport  Port=25
  OUT_26_manualToAutoHeight : Outport  Port=26
  OUT_27_finalApproachDistance : Outport  Port=27
  OUT_28_spreaderSwayAngle : Outport  Port=28
  OUT_29_spreaderSwayRate : Outport  Port=29
  OUT_30_scanProfileReq : Outport  Port=30
  OUT_31_lidarX : Outport  Port=31
  OUT_32_lidarY : Outport  Port=32
  OUT_33_scanSpeed : Outport  Port=33
  wires:
  IN_01_cmdStart/1 -> OUT_01_cmdStart/1
  IN_02_cmdStop/1 -> OUT_02_cmdStop/1
  IN_03_modeAutoReq/1 -> OUT_03_modeAutoReq/1
  IN_04_cmdAutoStart/1 -> OUT_04_cmdAutoStart/1
  IN_05_cmdReset/1 -> OUT_05_cmdReset/1
  IN_06_swayControlSelect/1 -> OUT_06_swayControlSelect/1
  IN_07_configValid/1 -> OUT_07_configValid/1
  IN_08_twistlockButton/1 -> OUT_08_twistlockButton/1
  IN_09_contact4/1 -> OUT_09_contact4/1
  IN_10_twistlocksClosedFb/1 -> OUT_10_twistlocksClosedFb/1
  IN_11_normalLimitXMin/1 -> OUT_11_normalLimitXMin/1
  IN_12_normalLimitXMax/1 -> OUT_12_normalLimitXMax/1
  IN_13_safetyPermitGlobal/1 -> OUT_13_safetyPermitGlobal/1
  IN_14_safetyPermitTrolley/1 -> OUT_14_safetyPermitTrolley/1
  IN_15_safetyPermitHoist/1 -> OUT_15_safetyPermitHoist/1
  IN_16_joyTrolley/1 -> OUT_16_joyTrolley/1
  IN_17_joyHoist/1 -> OUT_17_joyHoist/1
  IN_18_xTrolley/1 -> OUT_18_xTrolley/1
  IN_19_omegaTrolley/1 -> OUT_19_omegaTrolley/1
  IN_20_yHoist/1 -> OUT_20_yHoist/1
  IN_21_vHoist/1 -> OUT_21_vHoist/1
  IN_22_ropeTension/1 -> OUT_22_ropeTension/1
  IN_23_torqueTrolleyRaw/1 -> OUT_23_torqueTrolleyRaw/1
  IN_24_torqueHoistRaw/1 -> OUT_24_torqueHoistRaw/1
  IN_25_autoTargetX/1 -> OUT_25_autoTargetX/1
  IN_26_manualToAutoHeight/1 -> OUT_26_manualToAutoHeight/1
  IN_27_finalApproachDistance/1 -> OUT_27_finalApproachDistance/1
  IN_28_spreaderSwayAngle/1 -> OUT_28_spreaderSwayAngle/1
  IN_29_spreaderSwayRate/1 -> OUT_29_spreaderSwayRate/1
  IN_30_scanProfileReq/1 -> OUT_30_scanProfileReq/1
  IN_31_lidarX/1 -> OUT_31_lidarX/1
  IN_32_lidarY/1 -> OUT_32_lidarY/1
  IN_33_scanSpeed/1 -> OUT_33_scanSpeed/1

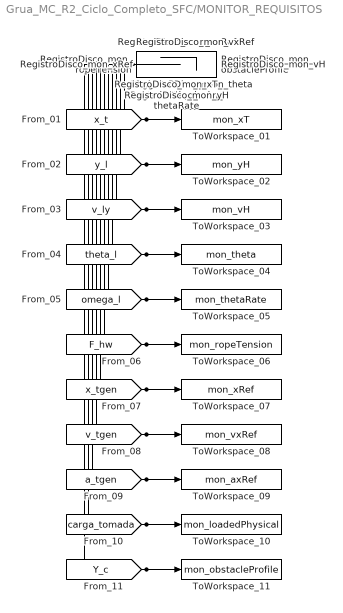
== system Grua_MC_R2_Ciclo_Completo_SFC/MONITOR_REQUISITOS ==
  RegistroDisco_mon_axRef : Terminator
  RegistroDisco_mon_loadedPhysical : Terminator
  RegistroDisco_mon_obstacleProfile : Terminator
  RegistroDisco_mon_ropeTension : Terminator
  RegistroDisco_mon_theta : Terminator
  RegistroDisco_mon_thetaRate : Terminator
  RegistroDisco_mon_vH : Terminator
  RegistroDisco_mon_vxRef : Terminator
  RegistroDisco_mon_xRef : Terminator
  RegistroDisco_mon_xT : Terminator
  RegistroDisco_mon_yH : Terminator
  ToWorkspace_01 : ToWorkspace  VariableName=mon_xT  SaveFormat=Timeseries  SampleTime=-1
  ToWorkspace_02 : ToWorkspace  VariableName=mon_yH  SaveFormat=Timeseries  SampleTime=-1
  ToWorkspace_03 : ToWorkspace  VariableName=mon_vH  SaveFormat=Timeseries  SampleTime=-1
  ToWorkspace_04 : ToWorkspace  VariableName=mon_theta  SaveFormat=Timeseries  SampleTime=-1
  ToWorkspace_05 : ToWorkspace  VariableName=mon_thetaRate  SaveFormat=Timeseries  SampleTime=-1
  ToWorkspace_06 : ToWorkspace  VariableName=mon_ropeTension  SaveFormat=Timeseries  SampleTime=-1
  ToWorkspace_07 : ToWorkspace  VariableName=mon_xRef  SaveFormat=Timeseries  SampleTime=-1
  ToWorkspace_08 : ToWorkspace  VariableName=mon_vxRef  SaveFormat=Timeseries  SampleTime=-1
  ToWorkspace_09 : ToWorkspace  VariableName=mon_axRef  SaveFormat=Timeseries  SampleTime=-1
  ToWorkspace_10 : ToWorkspace  VariableName=mon_loadedPhysical  SaveFormat=Timeseries  SampleTime=-1
  ToWorkspace_11 : ToWorkspace  VariableName=mon_obstacleProfile  SaveFormat=Timeseries  SampleTime=-1
  wires:
  [x_t] -> ToWorkspace_01/1, RegistroDisco_mon_xT/1
  [y_l] -> ToWorkspace_02/1, RegistroDisco_mon_yH/1
  [v_ly] -> ToWorkspace_03/1, RegistroDisco_mon_vH/1
  [theta_l] -> ToWorkspace_04/1, RegistroDisco_mon_theta/1
  [omega_l] -> ToWorkspace_05/1, RegistroDisco_mon_thetaRate/1
  [F_hw] -> ToWorkspace_06/1, RegistroDisco_mon_ropeTension/1
  [x_tgen] -> ToWorkspace_07/1, RegistroDisco_mon_xRef/1
  [v_tgen] -> ToWorkspace_08/1, RegistroDisco_mon_vxRef/1
  [a_tgen] -> ToWorkspace_09/1, RegistroDisco_mon_axRef/1
  [carga_tomada] -> ToWorkspace_10/1, RegistroDisco_mon_loadedPhysical/1
  [Y_c] -> ToWorkspace_11/1, RegistroDisco_mon_obstacleProfile/1

== system Grua_MC_R2_Ciclo_Completo_SFC/Motion Controller ==
  Sensors : Inport  OutDataTypeStr=Bus: MCFF_Sensors
  References : Inport  Port=2  OutDataTypeStr=Bus: MCFF_References
  Commands : Inport  Port=3  OutDataTypeStr=Bus: MCFF_Commands
  Drive Feedback : Inport  Port=4  OutDataTypeStr=Bus: MCFF_DriveFeedback
  Diagnosticos : Subsystem
  Estimadores : MATLAB Function  TreatAsAtomicUnit=on
  MC Carro : MATLAB Function  TreatAsAtomicUnit=on
  MC Izaje : MATLAB Function  TreatAsAtomicUnit=on
  Parameters : Constant  Value=MC_FF  OutDataTypeStr=Bus: MCFF_Parameters  SampleTime=T_s
  RegistroDisco_torque_carro_consigna_controlador : Terminator
  RegistroDisco_torque_izaje_consigna_controlador : Terminator
  RegistroPersistente_666 : ToWorkspace  VariableName=torque_carro_consigna_controlador  SaveFormat=Timeseries  SampleTime=-1
      settings: Decimation=10
  RegistroPersistente_667 : ToWorkspace  VariableName=antisway_efectiva  SaveFormat=Timeseries  SampleTime=-1
      settings: Decimation=10
  RegistroPersistente_668 : ToWorkspace  VariableName=diagnosticos_carro  SaveFormat=Timeseries  SampleTime=-1
      settings: Decimation=10
  RegistroPersistente_669 : ToWorkspace  VariableName=torque_izaje_consigna_controlador  SaveFormat=Timeseries  SampleTime=-1
      settings: Decimation=10
  RegistroPersistente_670 : ToWorkspace  VariableName=diagnosticos_izaje  SaveFormat=Timeseries  SampleTime=-1
      settings: Decimation=10
  T_hm* : Outport
  T_tmcontrolador : Outport  Port=2
  SW aplicada comun : Outport  Port=3
  Estados carro : Outport  Port=4
  Estados izaje : Outport  Port=5
  Diagnosticos carro : Outport  Port=6
  Diagnosticos izaje : Outport  Port=7
  wires:
  MC Carro/1(torque) -> T_tmcontrolador/1, RegistroPersistente_666/1, RegistroDisco_torque_carro_consigna_controlador/1
  Sensors/1 -> MC Carro/1(s), MC Izaje/1(s), Estimadores/1(s)
  Parameters/1 -> MC Carro/7(p), MC Izaje/4(p), Estimadores/2(p)
  MC Carro/2(sw) -> SW aplicada comun/1, RegistroPersistente_667/1
  Commands/1 -> MC Carro/3(c)
  Drive Feedback/1 -> MC Carro/4(drive)
  Estimadores/1(cart) -> MC Carro/5(est), Estados carro/1
  References/1 -> MC Carro/2(r), MC Izaje/2(r)
  Estimadores/2(hoist) -> MC Izaje/3(est), MC Carro/6(hoist), Estados izaje/1
  MC Carro/3(d) -> Diagnosticos/1(In1), Diagnosticos carro/1, RegistroPersistente_668/1
  MC Izaje/1(torque) -> T_hm*/1, RegistroPersistente_669/1, RegistroDisco_torque_izaje_consigna_controlador/1
  MC Izaje/2(d) -> Diagnosticos izaje/1, Diagnosticos/2(In2), RegistroPersistente_670/1

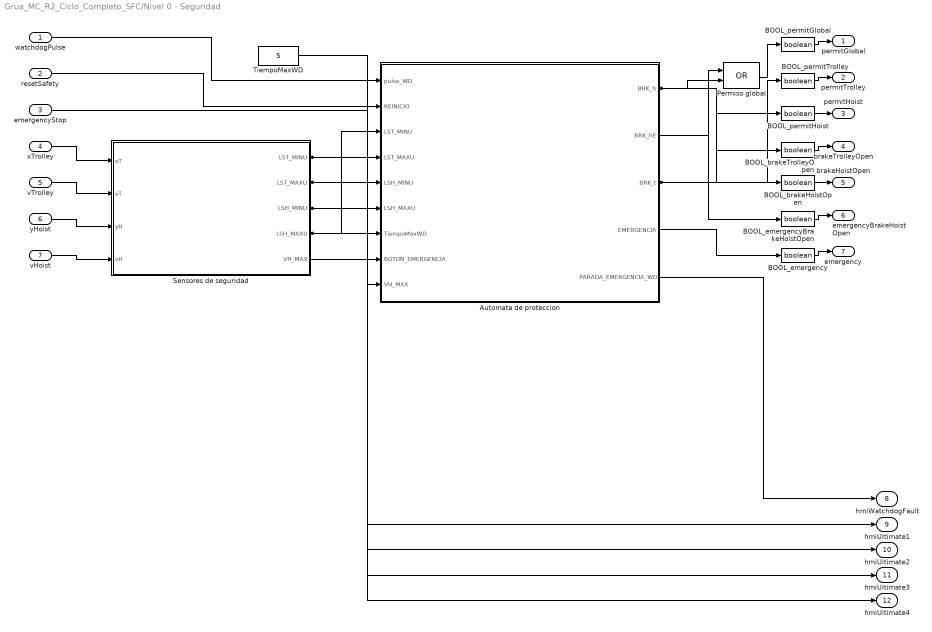
== system Grua_MC_R2_Ciclo_Completo_SFC/Nivel 0 - Seguridad ==
  watchdogPulse : Inport
  resetSafety : Inport  Port=2
  emergencyStop : Inport  Port=3
  xTrolley : Inport  Port=4
  vTrolley : Inport  Port=5
  yHoist : Inport  Port=6
  vHoist : Inport  Port=7
  Automata de proteccion : Subsystem
  BOOL_brakeHoistOpen : DataTypeConversion  OutDataTypeStr=boolean  SaturateOnIntegerOverflow=off  RndMeth=Floor
  BOOL_brakeTrolleyOpen : DataTypeConversion  OutDataTypeStr=boolean  SaturateOnIntegerOverflow=off  RndMeth=Floor
  BOOL_emergency : DataTypeConversion  OutDataTypeStr=boolean  SaturateOnIntegerOverflow=off  RndMeth=Floor
  BOOL_emergencyBrakeHoistOpen : DataTypeConversion  OutDataTypeStr=boolean  SaturateOnIntegerOverflow=off  RndMeth=Floor
  BOOL_permitGlobal : DataTypeConversion  OutDataTypeStr=boolean  SaturateOnIntegerOverflow=off  RndMeth=Floor
  BOOL_permitHoist : DataTypeConversion  OutDataTypeStr=boolean  SaturateOnIntegerOverflow=off  RndMeth=Floor
  BOOL_permitTrolley : DataTypeConversion  OutDataTypeStr=boolean  SaturateOnIntegerOverflow=off  RndMeth=Floor
  Permiso global : Logic  Operator=OR  AllPortsSameDT=off  OutDataTypeStr=boolean
  Sensores de seguridad : MATLAB Function  TreatAsAtomicUnit=on
  TiempoMaxWD : Constant  Value=5  OutDataTypeStr=double
  permitGlobal : Outport
  permitTrolley : Outport  Port=2
  permitHoist : Outport  Port=3
  brakeTrolleyOpen : Outport  Port=4
  brakeHoistOpen : Outport  Port=5
  emergencyBrakeHoistOpen : Outport  Port=6
  emergency : Outport  Port=7
  hmiWatchdogFault : Outport  Port=8
  hmiUltimate1 : Outport  Port=9
  hmiUltimate2 : Outport  Port=10
  hmiUltimate3 : Outport  Port=11
  hmiUltimate4 : Outport  Port=12
  wires:
  xTrolley/1 -> Sensores de seguridad/1(xT)
  vTrolley/1 -> Sensores de seguridad/2(vT)
  yHoist/1 -> Sensores de seguridad/3(yH)
  vHoist/1 -> Sensores de seguridad/4(vH)
  Sensores de seguridad/1(LST_MINU) -> hmiUltimate1/1, Automata de proteccion/3(LST_MINU)
  Sensores de seguridad/2(LST_MAXU) -> hmiUltimate2/1, Automata de proteccion/4(LST_MAXU)
  Sensores de seguridad/3(LSH_MINU) -> hmiUltimate3/1, Automata de proteccion/5(LSH_MINU)
  Sensores de seguridad/4(LSH_MAXU) -> hmiUltimate4/1, Automata de proteccion/6(LSH_MAXU)
  Permiso global/1 -> BOOL_permitGlobal/1
  BOOL_permitGlobal/1 -> permitGlobal/1
  BOOL_permitTrolley/1 -> permitTrolley/1
  BOOL_permitHoist/1 -> permitHoist/1
  BOOL_brakeTrolleyOpen/1 -> brakeTrolleyOpen/1
  BOOL_brakeHoistOpen/1 -> brakeHoistOpen/1
  BOOL_emergencyBrakeHoistOpen/1 -> emergencyBrakeHoistOpen/1
  BOOL_emergency/1 -> emergency/1
  watchdogPulse/1 -> Automata de proteccion/1(pulso_WD)
  resetSafety/1 -> Automata de proteccion/2(REINICIO)
  TiempoMaxWD/1 -> Automata de proteccion/7(TiempoMaxWD)
  emergencyStop/1 -> Automata de proteccion/8(BOTON_EMERGENCIA)
  Sensores de seguridad/5(VH_MAX) -> Automata de proteccion/9(VH_MAX)
  Automata de proteccion/1(BRK_h) -> Permiso global/2, BOOL_permitHoist/1, BOOL_brakeHoistOpen/1
  Automata de proteccion/2(BRK_hE) -> BOOL_emergencyBrakeHoistOpen/1
  Automata de proteccion/3(BRK_t) -> Permiso global/1, BOOL_permitTrolley/1, BOOL_brakeTrolleyOpen/1
  Automata de proteccion/4(EMERGENCIA) -> BOOL_emergency/1
  Automata de proteccion/5(PARADA_EMERGENCIA_WD) -> hmiWatchdogFault/1

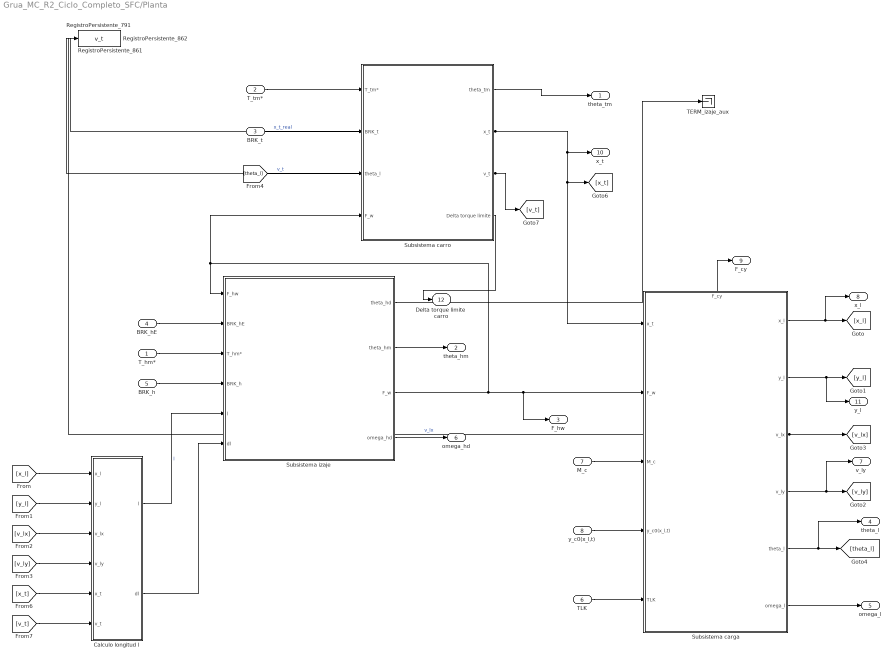
== system Grua_MC_R2_Ciclo_Completo_SFC/Planta ==
  T_hm* : Inport
  T_tm* : Inport  Port=2
  BRK_t : Inport  Port=3
  BRK_hE : Inport  Port=4
  BRK_h : Inport  Port=5
  TLK : Inport  Port=6
  M_c : Inport  Port=7
  y_c0(x_l,t) : Inport  Port=8
  Calculo longitud l : Subsystem
  RegistroPersistente_791 : ToWorkspace  VariableName=v_lx  SaveFormat=Timeseries  SampleTime=-1
      settings: Decimation=10
  RegistroPersistente_861 : ToWorkspace  VariableName=x_t_real  SaveFormat=Timeseries  SampleTime=-1
      settings: Decimation=10
  RegistroPersistente_862 : ToWorkspace  VariableName=v_t  SaveFormat=Timeseries  SampleTime=-1
      settings: Decimation=10
  Subsistema carga : Subsystem
      settings: PortSchema="{\"entries\":[{\"content\":{\"sides\":[{\"content\":{\"connectorIds\":[\"In1\",\"In2\",\"In3\",\"In4\",\"In5\"]},\"type\":\"ConnectorPlacement.EquallySpacedRectSide\",\"uuid\":\"47edabbd-243a-4b83-941f-e4392c1d00a7\"},{\"content\":{\"connectorIds\":[\"Out1\",\"Out2\",\"Out3\",\"Out4\",\"Out5\",\"Out6\"],\"side\":\"RIGHT\"},\"type\":\"ConnectorPlacement.EquallySpacedRectSide\",\"uuid\":\"f3c5bb4b-ba1f-46ef-b9da-f46dde7ba679\"},{\"content\":{\"connectorIds\":[\"Out7\"],\"side\":\"TOP\"},\"type\":\"ConnectorPlacement.EquallySpacedRectSide\",\"uuid\":\"99c64c8e-1061-494c-a8fc-4982bc564791\"}]},\"type\":\"ConnectorPlacement.EquallySpacedConnector\",\"uuid\":\"f8d59f7d-b4a0-41b3-9b68-cb1adbf574c0\"}],\"packageUris\":[\"http://schema.mathworks.com/mf0/Connector/R2020b\"],\"version\":\"1.0\"}"
  Subsistema carro : Subsystem
  Subsistema izaje : Subsystem
  TERM_izaje_aux : Terminator
  theta_tm : Outport
  theta_hm : Outport  Port=2
  F_hw : Outport  Port=3
  theta_l : Outport  Port=4
  omega_l : Outport  Port=5
  omega_hd : Outport  Port=6
  v_ly : Outport  Port=7
  x_l : Outport  Port=8
  F_cy : Outport  Port=9
  x_t : Outport  Port=10
  y_l : Outport  Port=11
  Delta torque limite carro : Outport  Port=12
  wires:
  y_c0(x_l,t)/1 -> Subsistema carga/4(y_c0(x_l,t))
  [x_t] -> Calculo longitud l/5(x_t)
  Subsistema izaje/3(F_w) -> Subsistema carro/4(F_w), Subsistema izaje/1(F_hw), F_hw/1, Subsistema carga/2(F_w)
  Subsistema carro/2(x_t) -> x_t/1, Subsistema carga/1(x_t), [x_t], RegistroPersistente_861/1  "x_t_real"
  [y_l] -> Calculo longitud l/2(y_l)
  BRK_hE/1 -> Subsistema izaje/2(BRK_hE)
  T_hm*/1 -> Subsistema izaje/3(T_hm*)
  T_tm*/1 -> Subsistema carro/1(T_tm*)
  Subsistema carga/3(v_lx) -> [v_lx], RegistroPersistente_791/1  "v_lx"
  [v_ly] -> Calculo longitud l/4(v_ly)
  Subsistema carga/2(y_l) -> [y_l], y_l/1
  Subsistema carga/4(v_ly) -> v_ly/1, [v_ly]
  Subsistema carga/1(x_l) -> x_l/1, [x_l]
  Subsistema carga/6(omega_l) -> omega_l/1
  [theta_l] -> Subsistema carro/3(theta_l)
  Calculo longitud l/2(dl) -> Subsistema izaje/6(dl)
  [v_lx] -> Calculo longitud l/3(v_lx)
  BRK_t/1 -> Subsistema carro/2(BRK_t)
  M_c/1 -> Subsistema carga/3(M_c)
  [x_l] -> Calculo longitud l/1(x_l)
  Subsistema carro/3(v_t) -> [v_t], RegistroPersistente_862/1  "v_t"
  Calculo longitud l/1(l) -> Subsistema izaje/5(l)  "l"
  [v_t] -> Calculo longitud l/6(v_t)
  BRK_h/1 -> Subsistema izaje/4(BRK_h)
  Subsistema izaje/4(omega_hd) -> omega_hd/1
  Subsistema carro/1(theta_tm) -> theta_tm/1
  Subsistema izaje/2(theta_hm) -> theta_hm/1
  Subsistema carga/5(theta_l) -> theta_l/1, [theta_l]
  Subsistema carga/7(F_cy) -> F_cy/1
  TLK/1 -> Subsistema carga/5(TLK)
  Subsistema izaje/1(theta_hd) -> TERM_izaje_aux/1
  Subsistema carro/4(Delta torque limite) -> Delta torque limite carro/1

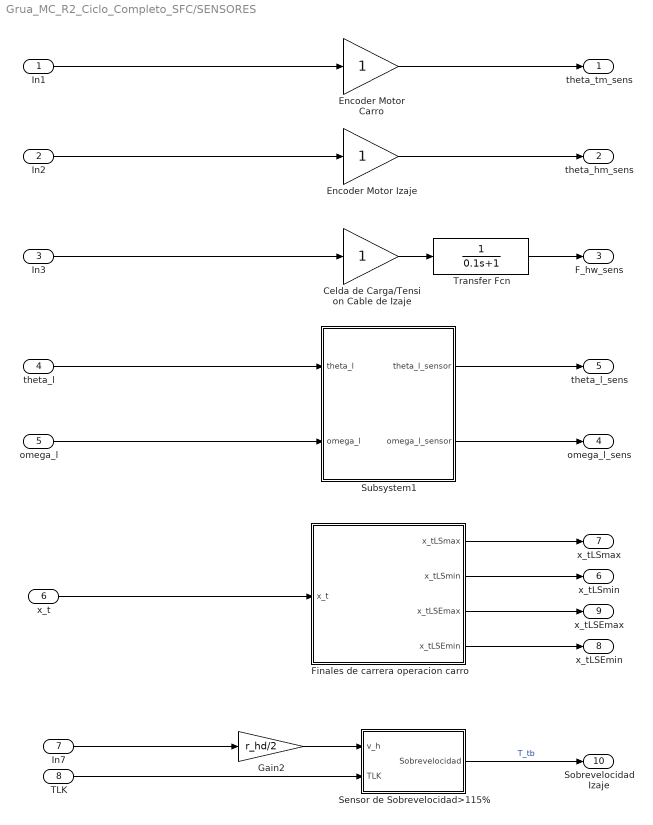
== system Grua_MC_R2_Ciclo_Completo_SFC/SENSORES ==
  In1 : Inport
  In2 : Inport  Port=2
  In3 : Inport  Port=3
  theta_l : Inport  Port=4
  omega_l : Inport  Port=5
  x_t : Inport  Port=6
  In7 : Inport  Port=7
  TLK : Inport  Port=8
  Celda de Carga/Tension Cable de Izaje : Gain
  Encoder Motor Carro : Gain
  Encoder Motor Izaje : Gain
  Finales de carrera operacion carro : Subsystem
  Gain2 : Gain  Gain=r_hd/2
  Sensor de Sobrevelocidad>115% : Subsystem
  Subsystem1 : Subsystem
  Transfer Fcn : TransferFcn  Denominator=[0.1 1]
  theta_tm_sens : Outport
  theta_hm_sens : Outport  Port=2
  F_hw_sens : Outport  Port=3
  omega_l_sens : Outport  Port=4
  theta_l_sens : Outport  Port=5
  x_tLSmin : Outport  Port=6
  x_tLSmax : Outport  Port=7
  x_tLSEmin : Outport  Port=8
  x_tLSEmax : Outport  Port=9
  Sobrevelocidad Izaje : Outport  Port=10
  wires:
  In1/1 -> Encoder Motor Carro/1
  Finales de carrera operacion carro/2(x_tLSmin) -> x_tLSmin/1
  Finales de carrera operacion carro/4(x_tLSEmin) -> x_tLSEmin/1
  Finales de carrera operacion carro/3(x_tLSEmax) -> x_tLSEmax/1
  Celda de Carga/Tension Cable de Izaje/1 -> Transfer Fcn/1
  Subsystem1/2(omega_l_sensor) -> omega_l_sens/1
  Encoder Motor Carro/1 -> theta_tm_sens/1
  Subsystem1/1(theta_l_sensor) -> theta_l_sens/1
  Sensor de Sobrevelocidad>115%/1(Sobrevelocidad) -> Sobrevelocidad Izaje/1  "T_tb"
  Gain2/1 -> Sensor de Sobrevelocidad>115%/1(v_h)
  x_t/1 -> Finales de carrera operacion carro/1(x_t)
  Encoder Motor Izaje/1 -> theta_hm_sens/1
  Finales de carrera operacion carro/1(x_tLSmax) -> x_tLSmax/1
  TLK/1 -> Sensor de Sobrevelocidad>115%/2(TLK)
  theta_l/1 -> Subsystem1/1(theta_l)
  In3/1 -> Celda de Carga/Tension Cable de Izaje/1
  omega_l/1 -> Subsystem1/2(omega_l)
  In2/1 -> Encoder Motor Izaje/1
  In7/1 -> Gain2/1
  Transfer Fcn/1 -> F_hw_sens/1

== system Grua_MC_R2_Ciclo_Completo_SFC/Subsystem1 ==
  Constant3 : Constant
  Demux : Demux  Outputs=6
  Gain11 : Gain  Gain=2
  Gain13 : Gain  Gain=-1
  Gain14 : Gain  Gain=-1
  Pilot Joystick All : aerolibanimutils/Pilot Joystick  JoystickID=None  OutputConfiguration=AllOutputs  SampleTime=1/3000
      settings: LibrarySourceBlock=aerolibanimutils/Pilot Joystick All
  RegistroPersistente_1113 : ToWorkspace  VariableName=joy_vert  SaveFormat=Timeseries  SampleTime=-1
      settings: Decimation=10
  RegistroPersistente_1114 : ToWorkspace  VariableName=joy_hor  SaveFormat=Timeseries  SampleTime=-1
      settings: Decimation=10
  RegistroPersistente_1115 : ToWorkspace  VariableName=analog  SaveFormat=Timeseries  SampleTime=-1
      settings: Decimation=10
  RegistroPersistente_1116 : ToWorkspace  VariableName=buttons  SaveFormat=Timeseries  SampleTime=-1
      settings: Decimation=10
  Sum5 : Sum  Inputs=|+-
  Terminator{8..12} (5 alike) : Terminator
  Transfer Fcn : TransferFcn  Denominator=[2 1]
  Transfer Fcn1 : TransferFcn  Denominator=[1 1]
  boton : Outport
  joy_vert : Outport  Port=2
  joy_hor : Outport  Port=3
  wires:
  Demux/5 -> Terminator10/1
  Pilot Joystick All/2 -> boton/1, RegistroPersistente_1116/1  "buttons"
  Demux/2 -> Transfer Fcn1/1
  Constant3/1 -> Sum5/2
  Pilot Joystick All/3 -> Terminator12/1  "POV"
  Transfer Fcn/1 -> Gain14/1
  Demux/1 -> Terminator8/1
  Sum5/1 -> Transfer Fcn/1
  Gain11/1 -> Sum5/1
  Demux/3 -> Gain11/1
  Transfer Fcn1/1 -> Gain13/1
  Pilot Joystick All/1 -> Demux/1, RegistroPersistente_1115/1  "analog"
  Demux/4 -> Terminator9/1
  Demux/6 -> Terminator11/1
  Gain14/1 -> joy_hor/1, RegistroPersistente_1114/1  "joy_hor"
  Gain13/1 -> joy_vert/1, RegistroPersistente_1113/1  "joy_vert"
